simulink model "bike_model"  (R2021a)
settings: Solver=VariableStepAuto  StartTime=0.0  StopTime=10.0  RelTol=1e-3
undefined symbols (not defined in the file or in its folder): A, B, C, D, sigbuilder_block
libraries: mpclib x1
settings Model: Creator=saksham  LastModifiedBy=saksham

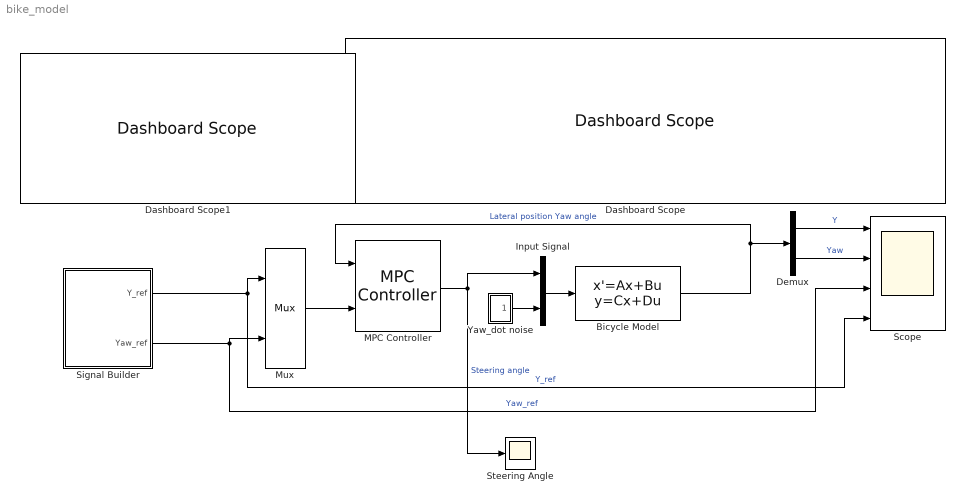
== system bike_model ==
  Bicycle Model : StateSpace  A=A  B=B  C=C  D=D  InitialCondition=[0,0,0,0]
  Dashboard Scope : DashboardScope
  Dashboard Scope1 : DashboardScope
  Demux : Demux  Outputs=2
  Input Signal : Mux  Inputs=2
  MPC Controller : mpclib/MPC Controller  SCDEnableBlockLinearizationSpecification=on  mpcobj=mpc1  is_multiple=0  enable_value=0  return_u0=off  updateMPCinCallerWorkspace=on  md_inport=off  mv_inport=off  uref_inport=off  return_cost=off  return_mvseq=off  return_qpstatus=off  return_xseq=off  return_state=off  return_ovseq=off  state_inport=off  umin_inport=off  umax_inport=off  ymin_inport=off  ymax_inport=off  cc_inport=off  ywt_inport=off  uwt_inport=off  duwt_inport=off  rhoeps_inport=off  pm_inport=off  MaximumP=10  HorizonChoice=FixedHorizon  n_ts=0.1  n_p=10  n_mv=1  n_md=0  n_ud=1  n_mo=2  n_uo=0  BlockDataType=double  SampleTimeInherited=off  switch_inport=off
  Mux : Mux  Inputs=2
      settings: DisplayOption=signals
  Scope : Scope  NumInputPorts=4
  Signal Builder : Subsystem  Tag=STV Subsys  LoadFcn=sigbuilder_block('load',[435 172 550 525 ]);  StartFcn=sigbuilder_block('start');  StopFcn=sigbuilder_block('stop');  ClipboardFcn=sigbuilder_block('clipboard');  mask(Sigbuilder block){tuvar=[0:10]}
      mask help: Simulink:masks:SigbuilderBlock_MD
      mask init:
      | if ~strcmp(get_param(bdroot(gcbh),'SimulationStatus'),'stopped') tuvar = sigbuilder_block('maskInit'); end
      settings: CopyFcn=sigbuilder_block('copy');  DeleteFcn=sigbuilder_block('delete');  ModelCloseFcn=sigbuilder_block('modelClose');  PreSaveFcn=sigbuilder_block('preSave');  PauseFcn=sigbuilder_block('pause');  ContinueFcn=sigbuilder_block('continue');  NameChangeFcn=sigbuilder_block('namechange');  OpenFcn=sigbuilder_block('open',[263 199 550 525 ]);  CloseFcn=sigbuilder_block('close');
      mask Display: plot(0, 0, 100, 100,[2, 2, 32, 32, 2], [68, 8, 8, 68, 68],[32, 2], [38, 38], [32, 19, 2],[53, 60, 44], [32, 17, 17, 2],[16, 16, 31, 31]);txt = getActiveGroup(gcbh);text(2, 100, txt,'verticalAlignment', 'top');
  "Steering Angle " : Scope
  Yaw_dot noise : Subsystem
  wires:
  MPC Controller/1 -> Input Signal/1, "Steering Angle "/1  "Steering angle"
  Bicycle Model/1 -> MPC Controller/1, Demux/1  "Lateral position Yaw angle"
  Mux/1 -> MPC Controller/2
  Signal Builder/2(Yaw_ref) -> Scope/3, Mux/2  "Yaw_ref"
  Demux/1 -> Scope/1  "Y"
  Demux/2 -> Scope/2  "Yaw"
  Signal Builder/1(Y_ref) -> Scope/4, Mux/1  "Y_ref"
  Input Signal/1 -> Bicycle Model/1
  Yaw_dot noise/1(Out1) -> Input Signal/2

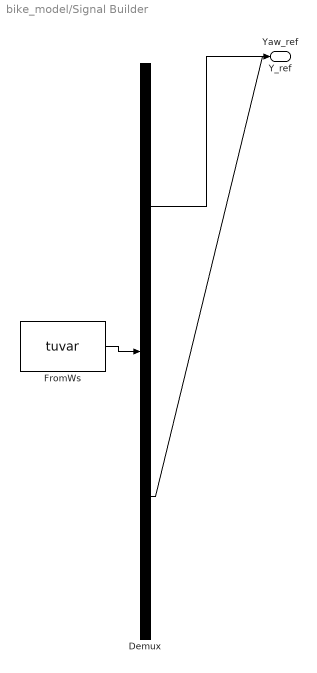
== system bike_model/Signal Builder ==
  Demux : Demux  Tag=STV Demux  Outputs=2
      settings: DisplayOption=none
  FromWs : FromWorkspace  Tag=STV FromWs  VariableName=tuvar
      SigBuilderData=|
      | common.afterFinalStr = 'Extrapolate'
      | common.sampleTime = 0
      | dataSet.timeRange = [0 10]
      | dataSet.name = 'Group 1'
      | sbobj.Groups.Name = 'Group 1'
      | sbobj.Groups.Signals(1).Name = 'Y_ref'
      | sbobj.Groups.Signals(1).XData = [0 1 2.95 2.95 6 6 10]
      | sbobj.Groups.Signals(1).YData = [0.5 0.5 1.5 1.49 1.5 1 0.5]
      | sbobj.Groups.Signals(2).Name = 'Yaw_ref'
      | sbobj.Groups.Signals(2).XData = [0 10]
      | sbobj.Groups.Signals(2).YData = [0 0]
  Y_ref : Outport  Tag=STV Outport
  Yaw_ref : Outport  Tag=STV Outport  Port=2
  wires:
  FromWs/1 -> Demux/1
  Demux/1 -> Y_ref/1
  Demux/2 -> Yaw_ref/1

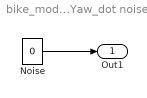
== system bike_model/Yaw_dot noise ==
  Noise : Constant  Value=0
  Out1 : Outport
  wires:
  Noise/1 -> Out1/1
